simulink model "simulation_ACC_test"  (R2018b)
settings: Solver=ode2  StartTime=0.0  StopTime=90  FixedStep=0.4  RelTol=1e-3
undefined symbols (not defined in the file or in its folder): Delta_T, DiscIntNeverNeededParam, lead_bot_vel_vari, lead_bot_vel_vari_const, sigbuilder_block, timebpt
libraries: commchan3 x11, visionstatistics x4, simulink x3
(part 3 of 3)

== matlab function simulation_ACC_test/1-D Kalman Filter3/MATLAB Function5 ==
  data: A input; K output; C input; Q input; R input; Pm input
% This code has referred from
% https://www.cs.cmu.edu/~cga/dynopt/kalman/kalman.html and
% https://statweb.stanford.edu/~candes/acm116/Handouts/Kalman.pdf
% for more info check it out.
% as we are having longitudinal autonomy, therefore taking simple state transition matrix!!
function K  = sim_vel_est_kalman_filt_1D(A, C, Q, R, Pm)
%{
    C = [1, 0];
R = [0.000225];
Q = [0.0001, 0;
      0, 0.0001];
P0 = [0.0001, 0;
       0, 0.0001];
    
sem = [0, 0]';
          if detectionClusters{1, 1}.Measurement(1, :) >= 0.5
            Q = [(0.035 * detectionClusters{1, 1}.Measurement(1, :))^2, 0;
                    0,  (0.035 * detectionClusters{1, 1}.Measurement(1, :))^2];
          end
          if detectionClusters{1, 1}.Measurement(1, :) >= 0.5
                R = [(0.05*detectionClusters{1, 1}.Measurement(1, :))^2];
          end
          if detectionClusters{1, 1}.Measurement(1, :) >= 0.5
                P0 = [(0.035 * detectionClusters{1, 1}.Measurement(1, :))^2, 0;
                        0 , (0.035 * detectionClusters{1, 1}.Measurement(1, :))^2];
          end
          dt = toc(tStart);
          tStart = tic;
          A = [1, dt;
                0, 1];
%}
% designing the Kalman filter

for i = 1:1000
% measurement step

    S = C * Pm * C' + R;
    %K = Pm*C'*inv(S); % change this inverse thing to solve with solutions of linear equations.
    % changing to linear eq solution:
    K =  Pm*C' * inv(S); % as it is 1 D dividing it, but for matrix linsolve is the best to get the "K".

    Pp = Pm - K*C*Pm;
 % prediction step
    Pm = A*Pp*A' + Q;
end

 
end

== matlab function simulation_ACC_test/MATLAB Function13 ==
  data: rel_velx input; accel_new output; rel_posx input; vel_egox input; stat output
function [accel_new, stat] = acc_sim(rel_velx, rel_posx, vel_egox)

%  MPC, solving QP problem: min (0.5*x'*H*x + f' * x) with
% linear inequality constraint A*x >= b
% speed: current speed
% accele_new: spit out the velocity of the turtlebot
% brake: stop while no movement of the lead vehicle vel_ego = accele_new =0.
% rel_dist : rel_posx distance between the ego and lead vehicle.
% vel_egox:  current speed of ego robot. this info will be
% taken from the imu of the vehicle/turtlebot.
% x_des: safe distance to be considered on the actual vehicle for braking
% is 0.4m in this case

% using reletive distance minimization.
% minimize J = |V - v_ego|^2
% const_vel = 0.02; % to keep the velocity of the turtlebot.
delta_t = 0.4;
x_des = 0.4; % minimum distance is 40 cm.
v_lead = rel_velx + vel_egox;
H = [2, 0; 
    0, 0.0001];
f= [-2*x_des; 0];
A = [0, 1;
    0, -1];
b = [0; -0.2];
iA0 = false(size(b));
Aeq = [1, delta_t];
%beq = rel_posx + Delta_T*Relatice_dis_deri + v_lead*delta_t;
beq = rel_posx + v_lead*delta_t;

[L,p] = chol(H,'lower');
Linv = inv(L);
%Linv = reshape(Linv,1,1);

opt = mpcqpsolverOptions;


%cold start the solver, inequality constraints
[x,stat,iA] = mpcqpsolver(Linv,f,A,b,Aeq,beq,iA0,opt);
if rel_velx < 0
    accel_new =0;
end

%if rel_velx > -0.2 & rel_velx < 0.2
    if stat > 0
     %if x ~= x_des
        %accel_new = rel_velx + vel_egox + const_vel;
     %
        accel_new =  x(2);
         
    else
           accel_new = vel_egox;
    end


% disp(['##1 -- Status : ',num2str(stat)])
% disp(['##2 -- relative position : ',num2str(rel_posx)])
% disp(['##2 -- ego velocity : ',num2str(vel_egox)])
% disp(['##2 -- relative velocity : ',num2str(rel_velx)])
% disp(['##2 -- Acceleration Command : ',num2str(accel_new)])
end

== matlab function simulation_ACC_test/New_1d_kalman_filter/MATLAB Function ==
  data: sem input; sensor_data input; sep output; A input; C input; Q input; R input; P0 input; sem output
function  [sep, sem] = new_kalman_sim_test(sem, sensor_data, A, C, Q, R, P0)
          if sensor_data(1) >= 0.5
            Q = [(0.035 * sensor_data(1))^2, 0;
                    0,  (0.035 * sensor_data(1))^2];
          end
          if sensor_data(1) >= 0.5
                R = [(0.05*sensor_data(1))^2];
          end
          if sensor_data(1) >= 0.5
                P0 = [(0.035 * sensor_data(1))^2, 0;
                        0 , (0.035 * sensor_data(1))^2];
          end
    Pm = P0;
    [K] = sim_vel_est_kalman_filt_1D( A, C, Q, R, Pm);
    sep = sem + K*(sensor_data(1) - C*sem);
    pose = [sep(1)];
    velex = [sep(2)];
          % prediction step
    sem = A*sep; %+ B*vele; % pass this final value

== matlab function simulation_ACC_test/New_1d_kalman_filter2/MATLAB Function ==
  data: sem input; sensor_data input; sep output; A input; C input; Q input; R input; P0 input; sem output
function  [sep, sem] = new_kalman_sim_test(sem, sensor_data, A, C, Q, R, P0)
          if sensor_data(1) >= 0.5
            Q = [(0.035 * sensor_data(1))^2, 0;
                    0,  (0.035 * sensor_data(1))^2];
          end
          if sensor_data(1) >= 0.5
                R = [(0.05*sensor_data(1))^2];
          end
          if sensor_data(1) >= 0.5
                P0 = [(0.035 * sensor_data(1))^2, 0;
                        0 , (0.035 * sensor_data(1))^2];
          end
    Pm = P0;
    [K] = sim_vel_est_kalman_filt_1D( A, C, Q, R, Pm);
    sep = sem + K*(sensor_data(1) - C*sem);
    pose = [sep(1)];
    velex = [sep(2)];
          % prediction step
    sem = A*sep; %+ B*vele; % pass this final value

== matlab function simulation_ACC_test/Sensor Fusion/New_1d_kalman_filter3/MATLAB Function ==
  data: sem input; sensor_data input; sep output; A input; C input; Q input; R input; P0 input; sem output
function  [sep, sem] = new_kalman_sim_test(sem, sensor_data, A, C, Q, R, P0)
          if sensor_data(1) >= 0.5
            Q = [(0.035 * sensor_data(1))^2, 0;
                    0,  (0.035 * sensor_data(1))^2];
          end
          if sensor_data(1) >= 0.5
                R = [(0.05*sensor_data(1))^2];
          end
          if sensor_data(1) >= 0.5
                P0 = [(0.035 * sensor_data(1))^2, 0;
                        0 , (0.035 * sensor_data(1))^2];
          end
    Pm = P0;
    [K] = sim_vel_est_kalman_filt_1D( A, C, Q, R, Pm);
    sep = sem + K*(sensor_data(1) - C*sem);
    pose = [sep(1)];
    velex = [sep(2)];
          % prediction step
    sem = A*sep; %+ B*vele; % pass this final value
